simulink library "discreteClampingPID"  (R2022a)
settings: Solver=VariableStepAuto  StartTime=0.0  StopTime=10.0  RelTol=1e-3
undefined symbols (not defined in the file): Ts
libraries: simulink x2, discreteFilter_ul x1
settings Model: Creator=adabney  LastModifiedBy=adabney

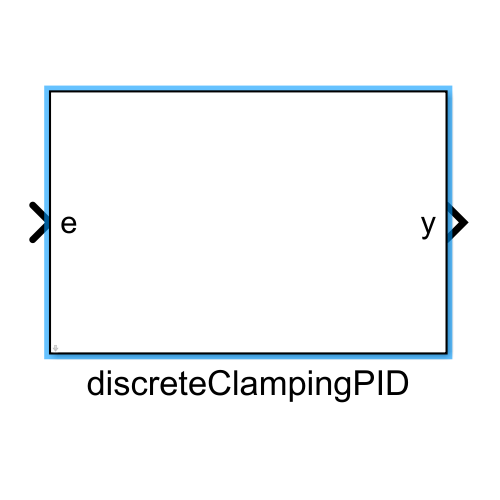
[thumbnail: Simulink's stored preview of the top-level diagram]
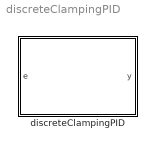
== system discreteClampingPID ==
  discreteClampingPID : Subsystem  mask{upperLim=0, lowerLim=0, kP=0, kI=0, kD=0, tau=0, Ts=Ts}
      mask prompts: upperLim "Upper Limit"; lowerLim "Lower Limit"; kP "Proportional Gain"; kI "Integral Gain"; kD "Derivative Gain"; tau "Filter Time Constant"; Ts "Sample Time"
      mask DialogControl DescTextVar Prompt: Discrete-time Filtered-PID Controller with Integral Clamping. When controller saturates, error signal feeding the integral is turned to zero to prevent integral wind up.
      mask DialogControl ParameterGroupVar Prompt: Controller Inputs
      mask DialogControl Container2 Prompt: Saturation Limits

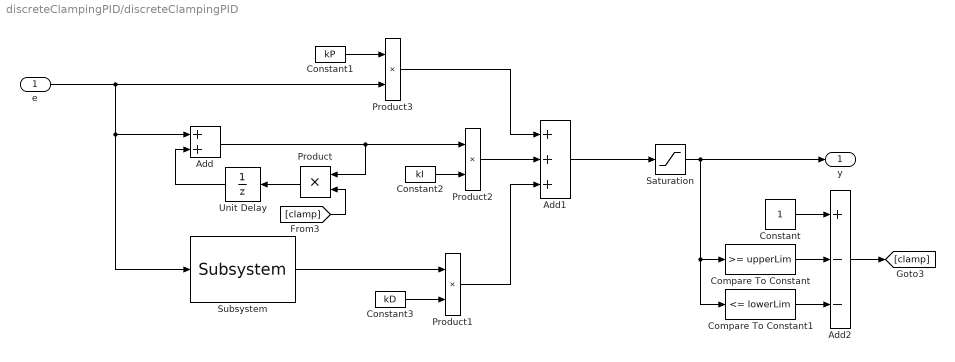
== system discreteClampingPID/discreteClampingPID ==
  e : Inport
  Add : Sum
  Add1 : Sum  Inputs=+++
  Add2 : Sum  Inputs=+--
  Compare To Constant : simulink/Logic and Bit Operations/Compare To Constant  relop=>=  const=upperLim  OutDataTypeStr=boolean
  Compare To Constant1 : simulink/Logic and Bit Operations/Compare To Constant  relop=<=  const=lowerLim  OutDataTypeStr=boolean
  Constant : Constant
  Constant1 : Constant  Value=kP
  Constant2 : Constant  Value=kI
  Constant3 : Constant  Value=kD
  Product{,1..3} (4 alike) : Product
  Saturation : Saturate  UpperLimit=upperLim  LowerLimit=lowerLim
  Subsystem : discreteFilter_ul/Subsystem  Ts=Ts  tau=tau
  Unit Delay : UnitDelay  SampleTime=-1  HasFrameUpgradeWarning=on
  y : Outport
  wires:
  Product1/1 -> Add1/3
  Add/1 -> Product/1, Product2/1
  Product3/1 -> Add1/1
  e/1 -> Product3/2, Subsystem/1, Add/1
  Constant3/1 -> Product1/2
  Constant2/1 -> Product2/2
  Constant1/1 -> Product3/1
  Add1/1 -> Saturation/1
  Product2/1 -> Add1/2
  Unit Delay/1 -> Add/2
  Subsystem/1 -> Product1/1
  Saturation/1 -> Compare To Constant1/1, Compare To Constant/1, y/1
  Compare To Constant1/1 -> Add2/3
  Compare To Constant/1 -> Add2/2
  Add2/1 -> [clamp]
  Product/1 -> Unit Delay/1
  [clamp] -> Product/2
  Constant/1 -> Add2/1
